simulink model "FOC_Model"  (R2020b)
settings: Solver=VariableStepAuto  StartTime=0.0  StopTime=10.0  RelTol=1e-3
undefined symbols (not defined in the file): B, Flux, J, Kt, Ls, Np, Rs, Udc
libraries: pid_lib x3, powerlib x1
settings Model: Creator=Administrator  LastModifiedBy=Administrator

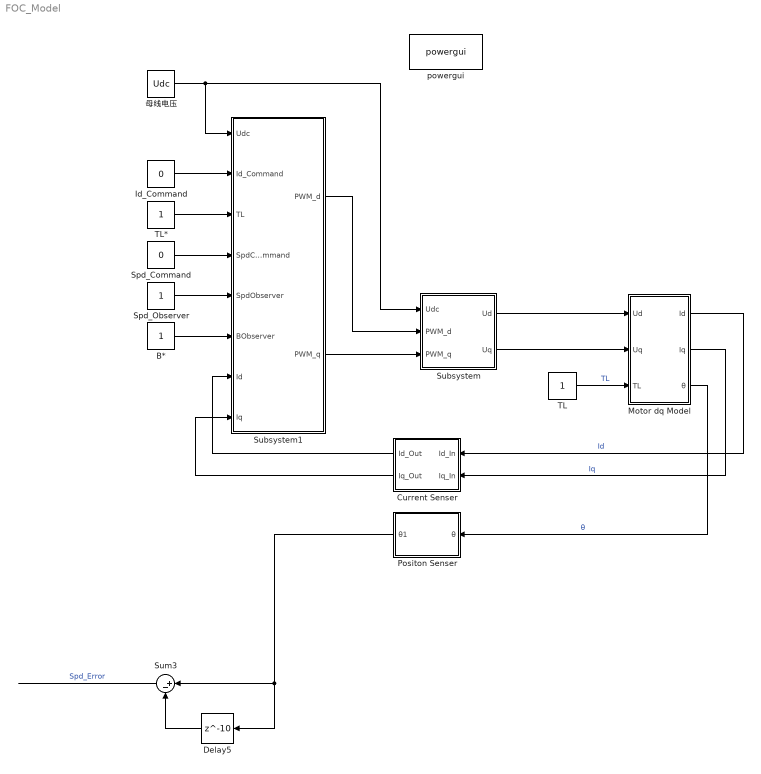
== system FOC_Model ==
  B* : Constant
  Current Senser : Subsystem
  Delay5 : Delay  DelayLength=10
  Id_Command : Constant  Value=0
  Motor dq Model : Subsystem
  Positon Senser : Subsystem
  Spd_Command : Constant  Value=0
  Spd_Observer : Constant
  Subsystem : Subsystem
  Subsystem1 : Subsystem
  Sum3 : Sum  Inputs=|+-
  TL : Constant
  TL* : Constant
  powergui : powerlib/powergui  Priority=1  SimulationMode=Discrete  SampleTime=1e-6  frequency=60  Iterations=50  frequencyindice=60  Pbase=100e6  ErrMax=1e-4  UnitsV=kV  UnitsW=MW  buscounter=0  FunctionMessages=off  echomessages=off  EnableUseOfTLC=off  CurrentSourceSwitches=off  DisableSnubberDevices=off  DisableRonSwitches=off  DisableVfSwitches=off  DisplayEquations=off  AutomaticDiscreteSolvers=off  SolverType=Tustin/Backward Euler (TBE)  Interpol=off  ExternalGateDelay=off  methode=off  Ts=100  x0status=blocks  SPID=on  SwTol=0  HookPort=off  NonlinearTolerance=1e-4  nMaxIteration=100  ContinueOnMaxIteration=off  RestoreLinks=warning  ResistiveCurrentMeasurement=off  Frange=[0:2:500]  Ylog=off  Xlog=on  ShowGrid=off  save=off  variable=ZData  structure=0  ZoomFFT=off  StartTime=0.0  cycles=1  DisplayStyle=1  fundamental=60  FreqAxis=off  MaxFrequency=1000  frequencyindicesteady=1  RmsSteady=1  display=off
  母线电压 : Constant  Value=Udc
  wires:
  Delay5/1 -> Sum3/2
  Sum3/1 -> ?  "Spd_Error"
  TL/1 -> Motor dq Model/3(TL)  "TL"
  Motor dq Model/1(Id) -> Current Senser/1(Id_In)  "Id"
  Motor dq Model/2(Iq) -> Current Senser/2(Iq_In)  "Iq"
  Positon Senser/1(θ1) -> Delay5/1, Sum3/1
  Motor dq Model/3(θ) -> Positon Senser/1(θ)  "θ"
  Subsystem/1(Ud) -> Motor dq Model/1(Ud)
  Subsystem/2(Uq) -> Motor dq Model/2(Uq)
  Id_Command/1 -> Subsystem1/2(Id_Command)
  TL*/1 -> Subsystem1/3(TL)
  Spd_Command/1 -> Subsystem1/4(SpdCommand)
  B*/1 -> Subsystem1/6(BObserver)
  Current Senser/1(Id_Out) -> Subsystem1/7(Id)
  Spd_Observer/1 -> Subsystem1/5(SpdObserver)
  Current Senser/2(Iq_Out) -> Subsystem1/8(Iq)
  Subsystem1/1(PWM_d) -> Subsystem/2(PWM_d)
  Subsystem1/2(PWM_q) -> Subsystem/3(PWM_q)
  母线电压/1 -> Subsystem/1(Udc), Subsystem1/1(Udc)

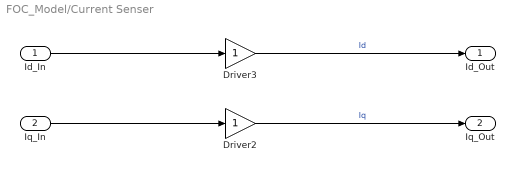
== system FOC_Model/Current Senser ==
  Id_In : Inport
  Iq_In : Inport  Port=2
  Driver2 : Gain
  Driver3 : Gain
  Id_Out : Outport
  Iq_Out : Outport  Port=2
  wires:
  Driver3/1 -> Id_Out/1  "Id"
  Id_In/1 -> Driver3/1
  Driver2/1 -> Iq_Out/1  "Iq"
  Iq_In/1 -> Driver2/1

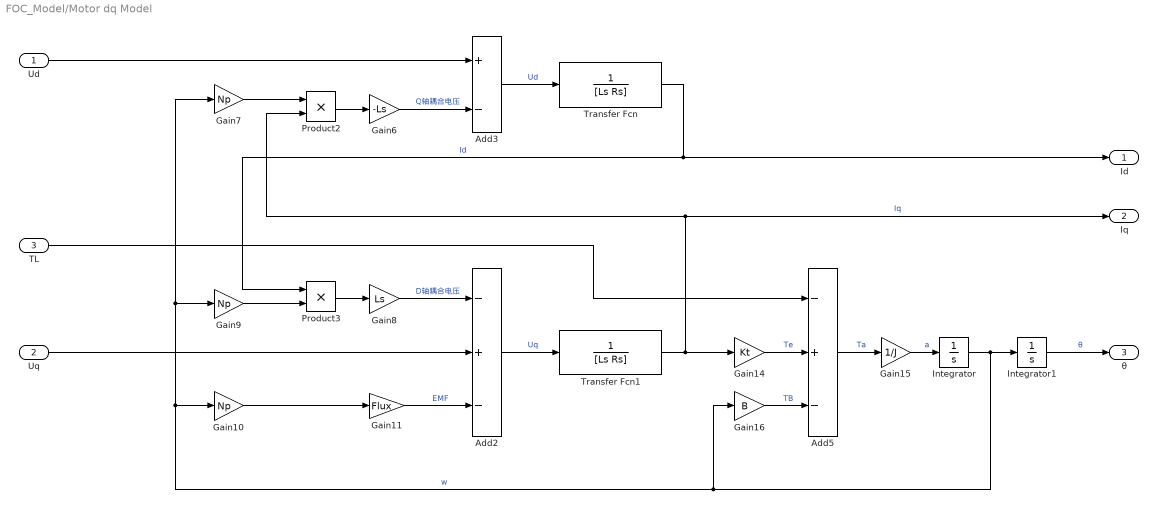
== system FOC_Model/Motor dq Model ==
  Ud : Inport
  Uq : Inport  Port=2
  TL : Inport  Port=3
  Add2 : Sum  Inputs=-+-
  Add3 : Sum  Inputs=+-
  Add5 : Sum  Inputs=-+-
  Gain10 : Gain  Gain=Np
  Gain11 : Gain  Gain=Flux
  Gain14 : Gain  Gain=Kt
  Gain15 : Gain  Gain=1/J
  Gain16 : Gain  Gain=B
  Gain6 : Gain  Gain=-Ls
  Gain7 : Gain  Gain=Np
  Gain8 : Gain  Gain=Ls
  Gain9 : Gain  Gain=Np
  Integrator : Integrator
  Integrator1 : Integrator
  Product2 : Product
  Product3 : Product
  Transfer Fcn : TransferFcn  Denominator=[Ls Rs]
  Transfer Fcn1 : TransferFcn  Denominator=[Ls Rs]
  Id : Outport
  Iq : Outport  Port=2
  θ : Outport  Port=3
  wires:
  Ud/1 -> Add3/1
  Product2/1 -> Gain6/1
  Add2/1 -> Transfer Fcn1/1  "Uq"
  Transfer Fcn1/1 -> Gain14/1, Product2/2, Iq/1  "Iq"
  Add3/1 -> Transfer Fcn/1  "Ud"
  Gain16/1 -> Add5/3  "TB"
  Transfer Fcn/1 -> Id/1, Product3/1  "Id"
  Product3/1 -> Gain8/1
  Gain9/1 -> Product3/2
  Gain14/1 -> Add5/2  "Te"
  Integrator/1 -> Gain16/1, Gain10/1, Gain7/1, Gain9/1, Integrator1/1  "w"
  Gain8/1 -> Add2/1  "D轴耦合电压"
  Gain6/1 -> Add3/2  "Q轴耦合电压"
  Gain7/1 -> Product2/1
  Gain10/1 -> Gain11/1
  Gain11/1 -> Add2/3  "EMF"
  Add5/1 -> Gain15/1  "Ta"
  Gain15/1 -> Integrator/1  "a"
  TL/1 -> Add5/1
  Uq/1 -> Add2/2
  Integrator1/1 -> θ/1  "θ"

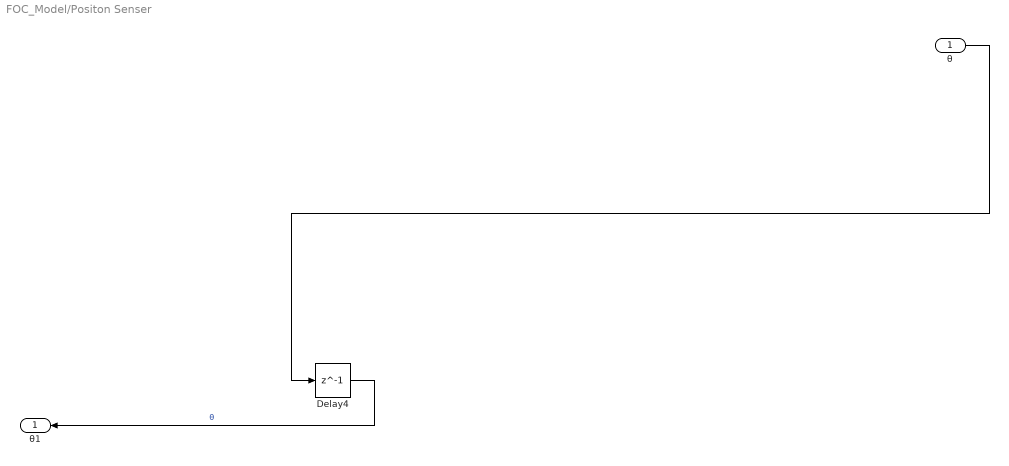
== system FOC_Model/Positon Senser ==
  θ : Inport
  Delay4 : Delay  DelayLength=1
  θ1 : Outport
  wires:
  Delay4/1 -> θ1/1  "θ"
  θ/1 -> Delay4/1

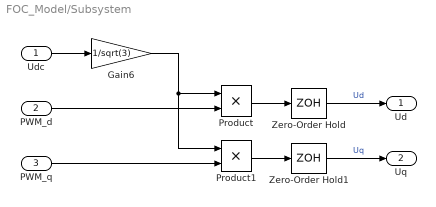
== system FOC_Model/Subsystem ==
  Udc : Inport
  PWM_d : Inport  Port=2
  PWM_q : Inport  Port=3
  Gain6 : Gain  Gain=1/sqrt(3)
  Product : Product
  Product1 : Product
  Zero-Order Hold : ZeroOrderHold  SampleTime=-1
  Zero-Order Hold1 : ZeroOrderHold  SampleTime=-1
  Ud : Outport
  Uq : Outport  Port=2
  wires:
  Product/1 -> Zero-Order Hold/1
  PWM_d/1 -> Product/2
  Zero-Order Hold1/1 -> Uq/1  "Uq"
  PWM_q/1 -> Product1/2
  Product1/1 -> Zero-Order Hold1/1
  Zero-Order Hold/1 -> Ud/1  "Ud"
  Udc/1 -> Gain6/1
  Gain6/1 -> Product/1, Product1/1

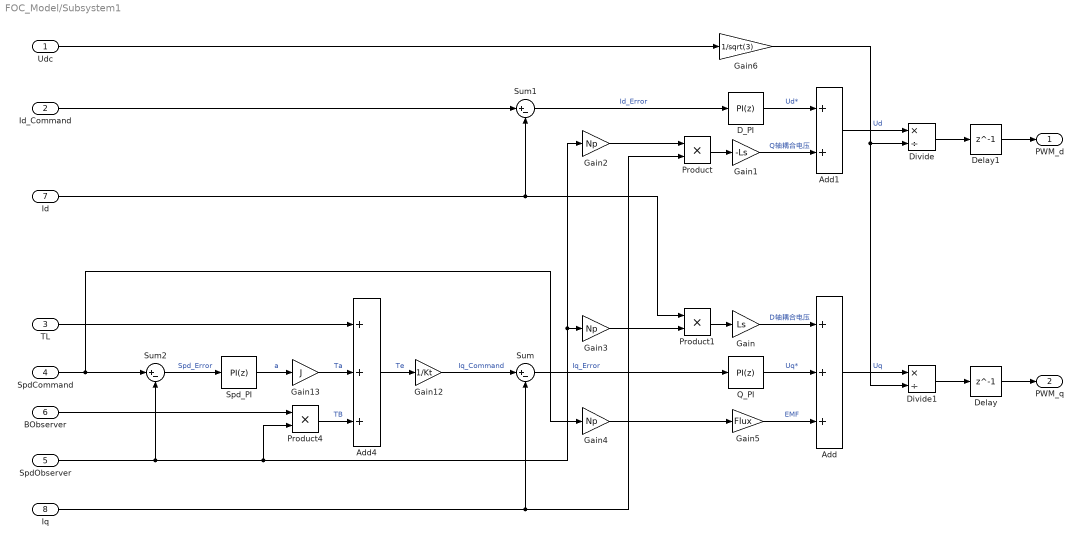
== system FOC_Model/Subsystem1 ==
  Udc : Inport
  Id_Command : Inport  Port=2
  TL : Inport  Port=3
  SpdCommand : Inport  Port=4
  SpdObserver : Inport  Port=5
  BObserver : Inport  Port=6
  Id : Inport  Port=7
  Iq : Inport  Port=8
  Add : Sum  Inputs=+++
  Add1 : Sum
  Add4 : Sum  Inputs=+++
  D_PI : pid_lib/PID Controller  Controller=PI  Form=Parallel  TimeDomain=Discrete-time  UseExternalTs=off  SampleTime=-1  IntegratorMethod=Forward Euler  FilterMethod=Forward Euler  ControllerParametersSource=internal  P=1  I=1  D=0  UseFilter=on  N=100  TunerSelectOption=Transfer Function Based (PID Tuner App)  InitialConditionSource=internal  InitialConditionForIntegrator=0  InitialConditionForFilter=0  DifferentiatorICPrevScaledInput=0  ExternalReset=none  TrackingMode=off  Kt=1  LimitOutput=off  SatLimitsSource=internal  UpperSaturationLimit=inf  LowerSaturationLimit=-inf  LinearizeAsGain=off  AntiWindupMode=none  Kb=1  POutMin=[]  POutMax=[]  IOutMin=[]  IOutMax=[]  DOutMin=[]  DOutMax=[]  NOutMin=[]  NOutMax=[]  SumOutMin=[]  SumOutMax=[]  SaturationOutMin=[]  SaturationOutMax=[]  PParamMin=[]  PParamMax=[]  IParamMin=[]  IParamMax=[]  DParamMin=[]  DParamMax=[]  NParamMin=[]  NParamMax=[]  KbParamMin=[]  KbParamMax=[]  KtParamMin=[]  KtParamMax=[]  KbOutMin=[]  KbOutMax=[]  KtOutMin=[]  KtOutMax=[]  IntegratorOutMin=[]  IntegratorOutMax=[]  FilterOutMin=[]  FilterOutMax=[]  SumI1OutMin=[]  SumI1OutMax=[]  SumI2OutMin=[]  SumI2OutMax=[]  SumI3OutMin=[]  SumI3OutMax=[]  SumI4OutMin=[]  SumI4OutMax=[]  SumDOutMin=[]  SumDOutMax=[]  DifferentiatorOutMin=[]  DifferentiatorOutMax=[]  FilterDiffOutCoefMin=[]  FilterDiffOutCoefMax=[]  ReciprocalOutMin=[]  ReciprocalOutMax=[]  SumDenOutMin=[]  SumDenOutMax=[]  SumNumOutMin=[]  SumNumOutMax=[]  DivideOutMin=[]  DivideOutMax=[]  UdiffTsProdOutMin=[]  UdiffTsProdOutMax=[]  NTsProdOutMin=[]  NTsProdOutMax=[]  UintegralTsProdOutMin=[]  UintegralTsProdOutMax=[]  UngainTsProdOutMin=[]  UngainTsProdOutMax=[]  IntegratorContinuousStateAttributes=''  IntegratorStateMustResolveToSignalObject=off  IntegratorRTWStateStorageClass=Auto  FilterContinuousStateAttributes=''  FilterStateMustResolveToSignalObject=off  FilterRTWStateStorageClass=Auto  ParallelPVariant=InternalParameters  IdealPVariant=Disabled  IVariant=InternalParameters  DVariant=Disabled  IntegratorVariant=Discrete  SatVariant=Disabled  AWVariant=Passthrough  PCopyVariant=Disabled  TRVariant=Disabled  FdbkBlocksVariant=Forward  IdealPFdbkVariant=Disabled  SatFdbkVariant=Disabled  DerivativeFilterVariant=Disabled  NVariant=Disabled  NCopyVariant=Disabled_SignalSpec  FilterICVariant=Disabled  IntegratorICVariant=InternalICs  ExternalResetVariant=Disabled  TRSumVariant=Passthrough  SumFdbkVariant=Disabled  SumVariant=Sum_PI  TsampFilterVariant=InternalTs  TsampNgainVariant=Passthrough  TsampIntegralVariant=Passthrough  ExternalSaturationOutDataTypeStr=Inherit: Same as second input
  Delay : Delay  DelayLength=1
  Delay1 : Delay  DelayLength=1
  Divide : Product  Inputs=*/
  Divide1 : Product  Inputs=*/
  Gain : Gain  Gain=Ls
  Gain1 : Gain  Gain=-Ls
  Gain12 : Gain  Gain=1/Kt
  Gain13 : Gain  Gain=J
  Gain2 : Gain  Gain=Np
  Gain3 : Gain  Gain=Np
  Gain4 : Gain  Gain=Np
  Gain5 : Gain  Gain=Flux
  Gain6 : Gain  Gain=1/sqrt(3)
  Product : Product
  Product1 : Product
  Product4 : Product
  Q_PI : pid_lib/PID Controller  Controller=PI  Form=Parallel  TimeDomain=Discrete-time  UseExternalTs=off  SampleTime=-1  IntegratorMethod=Forward Euler  FilterMethod=Forward Euler  ControllerParametersSource=internal  P=1  I=1  D=0  UseFilter=on  N=100  TunerSelectOption=Transfer Function Based (PID Tuner App)  InitialConditionSource=internal  InitialConditionForIntegrator=0  InitialConditionForFilter=0  DifferentiatorICPrevScaledInput=0  ExternalReset=none  TrackingMode=off  Kt=1  LimitOutput=off  SatLimitsSource=internal  UpperSaturationLimit=inf  LowerSaturationLimit=-inf  LinearizeAsGain=off  AntiWindupMode=none  Kb=1  POutMin=[]  POutMax=[]  IOutMin=[]  IOutMax=[]  DOutMin=[]  DOutMax=[]  NOutMin=[]  NOutMax=[]  SumOutMin=[]  SumOutMax=[]  SaturationOutMin=[]  SaturationOutMax=[]  PParamMin=[]  PParamMax=[]  IParamMin=[]  IParamMax=[]  DParamMin=[]  DParamMax=[]  NParamMin=[]  NParamMax=[]  KbParamMin=[]  KbParamMax=[]  KtParamMin=[]  KtParamMax=[]  KbOutMin=[]  KbOutMax=[]  KtOutMin=[]  KtOutMax=[]  IntegratorOutMin=[]  IntegratorOutMax=[]  FilterOutMin=[]  FilterOutMax=[]  SumI1OutMin=[]  SumI1OutMax=[]  SumI2OutMin=[]  SumI2OutMax=[]  SumI3OutMin=[]  SumI3OutMax=[]  SumI4OutMin=[]  SumI4OutMax=[]  SumDOutMin=[]  SumDOutMax=[]  DifferentiatorOutMin=[]  DifferentiatorOutMax=[]  FilterDiffOutCoefMin=[]  FilterDiffOutCoefMax=[]  ReciprocalOutMin=[]  ReciprocalOutMax=[]  SumDenOutMin=[]  SumDenOutMax=[]  SumNumOutMin=[]  SumNumOutMax=[]  DivideOutMin=[]  DivideOutMax=[]  UdiffTsProdOutMin=[]  UdiffTsProdOutMax=[]  NTsProdOutMin=[]  NTsProdOutMax=[]  UintegralTsProdOutMin=[]  UintegralTsProdOutMax=[]  UngainTsProdOutMin=[]  UngainTsProdOutMax=[]  IntegratorContinuousStateAttributes=''  IntegratorStateMustResolveToSignalObject=off  IntegratorRTWStateStorageClass=Auto  FilterContinuousStateAttributes=''  FilterStateMustResolveToSignalObject=off  FilterRTWStateStorageClass=Auto  ParallelPVariant=InternalParameters  IdealPVariant=Disabled  IVariant=InternalParameters  DVariant=Disabled  IntegratorVariant=Discrete  SatVariant=Disabled  AWVariant=Passthrough  PCopyVariant=Disabled  TRVariant=Disabled  FdbkBlocksVariant=Forward  IdealPFdbkVariant=Disabled  SatFdbkVariant=Disabled  DerivativeFilterVariant=Disabled  NVariant=Disabled  NCopyVariant=Disabled_SignalSpec  FilterICVariant=Disabled  IntegratorICVariant=InternalICs  ExternalResetVariant=Disabled  TRSumVariant=Passthrough  SumFdbkVariant=Disabled  SumVariant=Sum_PI  TsampFilterVariant=InternalTs  TsampNgainVariant=Passthrough  TsampIntegralVariant=Passthrough  ExternalSaturationOutDataTypeStr=Inherit: Same as second input
  Spd_PI : pid_lib/PID Controller  Controller=PI  Form=Parallel  TimeDomain=Discrete-time  UseExternalTs=off  SampleTime=-1  IntegratorMethod=Forward Euler  FilterMethod=Forward Euler  ControllerParametersSource=internal  P=1  I=1  D=0  UseFilter=on  N=100  TunerSelectOption=Transfer Function Based (PID Tuner App)  InitialConditionSource=internal  InitialConditionForIntegrator=0  InitialConditionForFilter=0  DifferentiatorICPrevScaledInput=0  ExternalReset=none  TrackingMode=off  Kt=1  LimitOutput=off  SatLimitsSource=internal  UpperSaturationLimit=inf  LowerSaturationLimit=-inf  LinearizeAsGain=off  AntiWindupMode=none  Kb=1  POutMin=[]  POutMax=[]  IOutMin=[]  IOutMax=[]  DOutMin=[]  DOutMax=[]  NOutMin=[]  NOutMax=[]  SumOutMin=[]  SumOutMax=[]  SaturationOutMin=[]  SaturationOutMax=[]  PParamMin=[]  PParamMax=[]  IParamMin=[]  IParamMax=[]  DParamMin=[]  DParamMax=[]  NParamMin=[]  NParamMax=[]  KbParamMin=[]  KbParamMax=[]  KtParamMin=[]  KtParamMax=[]  KbOutMin=[]  KbOutMax=[]  KtOutMin=[]  KtOutMax=[]  IntegratorOutMin=[]  IntegratorOutMax=[]  FilterOutMin=[]  FilterOutMax=[]  SumI1OutMin=[]  SumI1OutMax=[]  SumI2OutMin=[]  SumI2OutMax=[]  SumI3OutMin=[]  SumI3OutMax=[]  SumI4OutMin=[]  SumI4OutMax=[]  SumDOutMin=[]  SumDOutMax=[]  DifferentiatorOutMin=[]  DifferentiatorOutMax=[]  FilterDiffOutCoefMin=[]  FilterDiffOutCoefMax=[]  ReciprocalOutMin=[]  ReciprocalOutMax=[]  SumDenOutMin=[]  SumDenOutMax=[]  SumNumOutMin=[]  SumNumOutMax=[]  DivideOutMin=[]  DivideOutMax=[]  UdiffTsProdOutMin=[]  UdiffTsProdOutMax=[]  NTsProdOutMin=[]  NTsProdOutMax=[]  UintegralTsProdOutMin=[]  UintegralTsProdOutMax=[]  UngainTsProdOutMin=[]  UngainTsProdOutMax=[]  IntegratorContinuousStateAttributes=''  IntegratorStateMustResolveToSignalObject=off  IntegratorRTWStateStorageClass=Auto  FilterContinuousStateAttributes=''  FilterStateMustResolveToSignalObject=off  FilterRTWStateStorageClass=Auto  ParallelPVariant=InternalParameters  IdealPVariant=Disabled  IVariant=InternalParameters  DVariant=Disabled  IntegratorVariant=Discrete  SatVariant=Disabled  AWVariant=Passthrough  PCopyVariant=Disabled  TRVariant=Disabled  FdbkBlocksVariant=Forward  IdealPFdbkVariant=Disabled  SatFdbkVariant=Disabled  DerivativeFilterVariant=Disabled  NVariant=Disabled  NCopyVariant=Disabled_SignalSpec  FilterICVariant=Disabled  IntegratorICVariant=InternalICs  ExternalResetVariant=Disabled  TRSumVariant=Passthrough  SumFdbkVariant=Disabled  SumVariant=Sum_PI  TsampFilterVariant=InternalTs  TsampNgainVariant=Passthrough  TsampIntegralVariant=Passthrough  ExternalSaturationOutDataTypeStr=Inherit: Same as second input
  Sum : Sum  Inputs=|+-
  Sum1 : Sum  Inputs=|+-
  Sum2 : Sum  Inputs=|+-
  PWM_d : Outport
  PWM_q : Outport  Port=2
  wires:
  Sum/1 -> Q_PI/1  "Iq_Error"
  Gain4/1 -> Gain5/1
  Q_PI/1 -> Add/2  "Uq*"
  Spd_PI/1 -> Gain13/1  "a"
  Id/1 -> Product1/1, Sum1/2
  Product1/1 -> Gain/1
  Sum1/1 -> D_PI/1  "Id_Error"
  Gain12/1 -> Sum/1  "Iq_Command"
  Product/1 -> Gain1/1
  Gain1/1 -> Add1/2  "Q轴耦合电压"
  Gain5/1 -> Add/3  "EMF"
  SpdObserver/1 -> Gain2/1, Gain3/1, Product4/2, Sum2/2
  Gain3/1 -> Product1/2
  D_PI/1 -> Add1/1  "Ud*"
  Gain/1 -> Add/1  "D轴耦合电压"
  Add4/1 -> Gain12/1  "Te"
  Gain2/1 -> Product/1
  Iq/1 -> Product/2, Sum/2
  Sum2/1 -> Spd_PI/1  "Spd_Error"
  Product4/1 -> Add4/3  "TB"
  SpdCommand/1 -> Gain4/1, Sum2/1
  Gain13/1 -> Add4/2  "Ta"
  TL/1 -> Add4/1
  Add1/1 -> Divide/1  "Ud"
  Id_Command/1 -> Sum1/1
  BObserver/1 -> Product4/1
  Add/1 -> Divide1/1  "Uq"
  Divide/1 -> Delay1/1
  Udc/1 -> Gain6/1
  Divide1/1 -> Delay/1
  Gain6/1 -> Divide1/2, Divide/2
  Delay1/1 -> PWM_d/1
  Delay/1 -> PWM_q/1
